simulink model "pe_asm_generator_2"  (R2016b)
settings: Solver=ode23t  StartTime=0.0  StopTime=336  MaxStep=1e-4  RelTol=1e-3  EnableMultiTasking=on
PreLoadFcn:
  | SRated = 150e3; % W
  | VRated = 440; % V
  | FRated = 60; % Hz
  | 
  | QNominal = sin(acos(0.8))*SRated;
  | QPerPhase = QNominal / 3;
  | 
  | IPerPhase = QPerPhase/VRated;
  | Xc = VRated/IPerPhase;
  | reactiveCompensationCapacitance = 1/(2*pi*FRated*Xc);
  | 
  | clear( 'QNominal', 'QPerPhase', 'IPerPhase', 'Xc' );
undefined symbols (not defined in the file or in its folder): pe
libraries: pe_lib x8, nesl_utility x4, fl_lib x2
Description:
  | Three-Phase Asynchronous Wind Turbine Generator
  | 
  | This example shows an induction machine used as a wind turbine generator.
  | The Simple Turbine block converts wind speed to turbine output power by a
  | simple output power versus wind speed characteristic.
  | 
  | When the wind speed is below the cut-in speed or above the cut-out speed,
  | the machine generates zero real power. The machine always consumes
  | reactive power. The Reactive Compensation block offsets the machine's
  | reactive power requirement.
  | 
  | The local load consumes 75kW. The infeed from the power grid meets any
  | wind turbine generation shortfall. When the generator produces more than
  | 75kW, excess power is exported to the grid.
  | 
  | 
  | Copyright 2008-2015 The MathWorks, Inc.
settings Model: Creator=MathWorks  LastModifiedBy=oka
settings DataIOCC: LimitDataPoints=on  SaveFormat=Array  SaveOutput=off  SignalLogging=off  DSMLogging=off  SaveTime=off
settings OptimizationCC: LifeSpan=inf
settings DebuggingCC: UnderspecifiedInitializationDetection=Classic  MergeDetectMultiDrivingBlocksExec=none  SFUnexpectedBacktrackingDiag=warning  SFNoUnconditionalDefaultTransitionDiag=warning  SFExecutionAtInitializationDiag=none
settings HardwareCC: ProdBitPerPointer=32  ProdBitPerSizeT=32  ProdBitPerPtrDiffT=32  ProdLargestAtomicFloat=None  ProdIntDivRoundTo=Undefined  ProdEndianess=Unspecified  ProdWordSize=32  ProdHWDeviceType=32-bit Generic
settings ModelReferenceCC: PropagateSignalLabelsOutOfModel=off
settings GRTTargetCC: TargetLangStandard=C89/C90 (ANSI)  GeneratePreprocessorConditionals=Disable all
settings ConfigComp: CovMetricSettings=dw  CovHtmlReporting=on  CovSaveCumulativeToWorkspaceVar=on  CovSaveSingleToWorkspaceVar=on  CovExternalEMLEnable=off  CovSFcnEnable=off
settings SimscapeCC: SimscapeLogSimulationStatistics=on  SimscapeLogOpenViewer=on  SimscapeLogLimitData=off

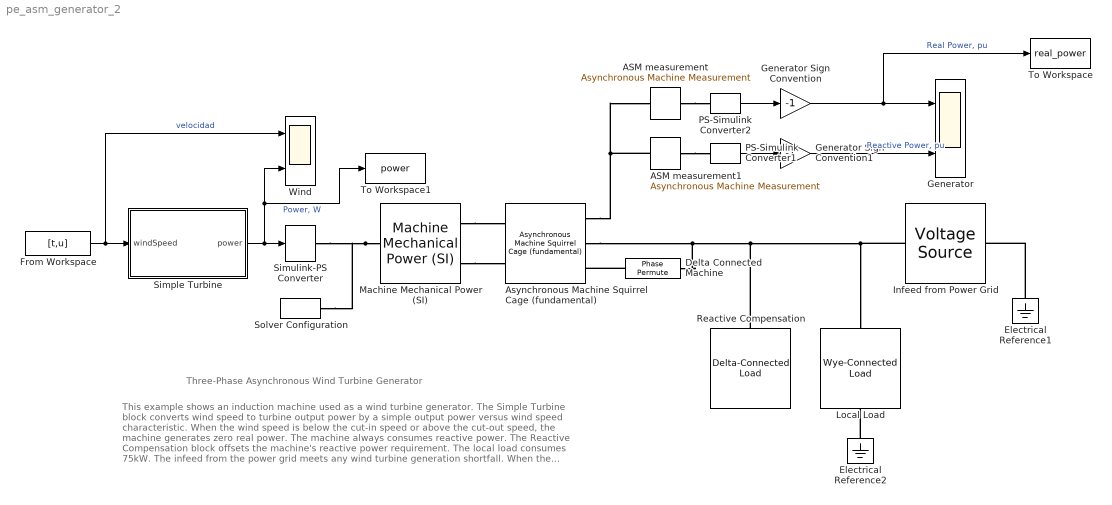
== system pe_asm_generator_2 ==
  note: This example shows an induction machine used as a wind turbine generator.  The Simple
      | Turbine block converts wind speed to turbine output power by a simple output power versus
      | wind speed characteristic.
      | When the wind speed is below the cut-in speed or above the cut-out speed, the machine
      | generates zero real power. The machine always consumes reactive power. The Reactive
      | Compensation block offsets the machine's reactive power requirement.
      | The local load consumes 75kW. The infeed from the power grid meets any wind turbine
      | generation shortfall. When the generator produces more than 75kW, excess power is
      | exported to the grid.
  note: Three-Phase Asynchronous Wind Turbine Generator
  ASM measurement : pe_lib/Machines/Asynchronous Machine Measurement  output_idx=11
  ASM measurement1 : pe_lib/Machines/Asynchronous Machine Measurement  output_idx=12
  Asynchronous Machine Squirrel Cage (fundamental) : pe_lib/Machines/Asynchronous Machine (Squirrel Cage)/Asynchronous Machine Squirrel Cage (fundamental)  SRated=SRated V*A  VRated=VRated V  FRated=FRated Hz  nPolePairs=2  Rs=0.0258  Lls=0.0930  Rrd=0.0145  Llrd=0.0424  Lm=1.7562  L0=0.0930  angular_position0=0 deg  pu_psids0=0  pu_psiqs0=0  pu_psi0s0=0  pu_psidr0=0  pu_psiqr0=0  oneOverOmega=nan s/rad  Lss=nan  Lrrd=nan  shift_3ph=[nan, nan, nan] rad  connection_option=int32(pe.Connection.delta)  base_v=nan V  base_i=nan A  base_torque=nan N*m  base_wMechanical=nan rad/s  base_wElectrical=nan rad/s
  Delta Connected Machine : pe_lib/Connections/Phase Permute
  Electrical Reference1 : fl_lib/Electrical/Electrical Elements/Electrical Reference
  Electrical Reference2 : fl_lib/Electrical/Electrical Elements/Electrical Reference
  From Workspace : FromWorkspace  VariableName=[t,u]  SampleTime=0
  Generator : Scope  NumInputPorts=2
  Generator Sign Convention : Gain  Gain=-1
  Generator Sign Convention1 : Gain  Gain=-1
  Infeed from Power Grid : pe_lib/Sources/Voltage Source  vline_rms=VRated V  shift=0 deg  freq=FRated Hz  harmonic_option=0  harmonic_orders=[5, 7, 11, 13]  harmonic_ratios=[0.1, 0.1, 0.1, 0.1]
  Local Load : pe_lib/Passive Devices/Wye-Connected Load  parameterization=2  component_structure=1  component_structure_PQ=1  R=1 Ohm  L=0.001 H  C=1e-6 F  IL0=[ 0 0 0 ] A  VC0=[ 0 0 0 ] V  R_parasitic=1e-6 Ohm  G_parasitic=1e-6 1/Ohm  VRated=VRated V  FRated=60 Hz  P=75e3 W  Qpos=100 V*A  Qneg=-100 V*A  Vmag0=2.4e+4 V  Vang0=0 deg  Freq0=60 Hz  R_parasitic_PQ=1e-6 Ohm  G_parasitic_PQ=1e-6 1/Ohm
  Machine Mechanical Power (SI) : pe_lib/Machines/Machine Mechanical Power (SI)  power_sign=-1  SRated=SRated V*A  FRated=FRated Hz  nPolePairs=2  torque_factor=2  inertia_option=2  J=27548 kg*m^2  H=4 s*W/V/A  damper_option=2  D=39.0509 N*m/(rad/s)  pu_D=0.01  initialization_option=2  fMechanical0=30 Hz  fElectrical0=FRated Hz
  PS-Simulink Converter1 : nesl_utility/PS-Simulink Converter  PhysicalDomain=network_engine_domain  SubClassName=ps_output  LeftPortType=input  RightPortType=output  PseudoPeriodic=off  Frequencies=[]  Unit=1  AffineConversion=off
  PS-Simulink Converter2 : nesl_utility/PS-Simulink Converter  PhysicalDomain=network_engine_domain  SubClassName=ps_output  LeftPortType=input  RightPortType=output  PseudoPeriodic=off  Frequencies=[]  Unit=1  AffineConversion=off
  Reactive Compensation : pe_lib/Passive Devices/Delta-Connected Load  parameterization=1  component_structure=3  component_structure_PQ=1  R=1 Ohm  L=0.001 H  C=reactiveCompensationCapacitance F  IL0=[ 0 0 0 ] A  VC0=[ 0 0 0 ] V  R_parasitic=1e-6 Ohm  G_parasitic=1e-6 1/Ohm  VRated=2.4e+4 V  FRated=60 Hz  P=1000 W  Qpos=100 V*A  Qneg=-100 V*A  Vmag0=2.4e+4 V  Vang0=0 deg  Freq0=60 Hz  R_parasitic_PQ=1e-6 Ohm  G_parasitic_PQ=1e-6 1/Ohm
  Simple Turbine : MATLAB Function  TreatAsAtomicUnit=on  mask(Simple Turbine){ratedOutputPower=150e3, cutInSpeed=3, ratedOutputSpeed=12, cutOutSpeed=23}
      mask prompts: ratedOutputPower "Rated output power, W"; cutInSpeed "Cut-in speed, m/s"; ratedOutputSpeed "Rated output speed, m/s"; cutOutSpeed "Cut-out speed, m/s"
      mask help:
      | This function implements a simple power versus wind speed characteristic to represent a wind turbine.
      |
      | Given an input of wind speed, m/s, the function outputs turbine power, W.
      |
      | The parameters must meet the following requirement:
      |
      | Cut-in speed < Rated output speed < Cut-out speed
  Simulink-PS Converter : nesl_utility/Simulink-PS Converter  PhysicalDomain=network_engine_domain  SubClassName=ps_input  LeftPortType=input  RightPortType=output  PseudoPeriodic=off  Frequencies=[]  NoiseDistribution=none  NoiseParameters=[]  Unit=1  AffineConversion=off  InputFiltering=off  SimscapeFilterOrder=1  InputFilterTimeConstant=0.001  UdotUserProvided=1
  Solver Configuration : nesl_utility/Solver Configuration  PhysicalDomain=network_engine_domain  SubClassName=solver  LeftPortType=input  RightPortType=generic  Accelerate=off  Tones=[]  Harmonics=[]  SimulateNoise=off  Profile=off  UseLocalSampling=off  EnableSwitchedLinearOptims=on  FrequencyDomain=off  UseCCode=off  RelTol=0.001  AbsTol=1e-06  MinStep=1e-09  ToWorkspace=off  RevertToSquareIcSolve=off  NumHomotopyIterations=100  PhasorMode=off  PhasorModeNumHarmonics=1  OverrideAbsTol=off  DoDC=off  ResidualTolerance=1e-9  UseLocalSolver=on  LocalSolverChoice=NE_BACKWARD_EULER_ADVANCER  LocalSolverSampleTime=1e-3  DoFixedCost=on  MaxNonlinIter=3  MaxModeIter=2  LinearAlgebra=Sparse  DelaysMemoryBudget=1024  AutomaticFiltering=on  FilteringTimeConstant=0.001
  To Workspace : ToWorkspace  VariableName=real_power  SampleTime=-1
  To Workspace1 : ToWorkspace  VariableName=power  SampleTime=-1
  Wind : Scope  NumInputPorts=2
  wires:
  PS-Simulink Converter2/1 -> Generator Sign Convention/1
  PS-Simulink Converter1/1 -> Generator Sign Convention1/1
  Generator Sign Convention/1 -> To Workspace/1, Generator/1  "Real Power, pu"
  Generator Sign Convention1/1 -> Generator/2  "Reactive Power, pu"
  From Workspace/1 -> Simple Turbine/1(windSpeed), Wind/1  "velocidad"
  Simple Turbine/1(power) -> Simulink-PS Converter/1, To Workspace1/1, Wind/2  "Power, W"
  connections:
  Asynchronous Machine Squirrel Cage (fundamental)/RConn2 -- Reactive Compensation/LConn1 -- Infeed from Power Grid/RConn1 -- Local Load/LConn1 -- Delta Connected Machine/LConn1
  Machine Mechanical Power (SI)/RConn1 -- Asynchronous Machine Squirrel Cage (fundamental)/LConn1
  Machine Mechanical Power (SI)/RConn2 -- Asynchronous Machine Squirrel Cage (fundamental)/LConn2
  Machine Mechanical Power (SI)/LConn1 -- Solver Configuration/RConn1 -- Simulink-PS Converter/RConn1
  Asynchronous Machine Squirrel Cage (fundamental)/RConn1 -- ASM measurement1/LConn1 -- ASM measurement/LConn1
  ASM measurement/RConn1 -- PS-Simulink Converter2/LConn1
  Delta Connected Machine/RConn1 -- Asynchronous Machine Squirrel Cage (fundamental)/RConn3
  Electrical Reference1/LConn1 -- Infeed from Power Grid/LConn1
  ASM measurement1/RConn1 -- PS-Simulink Converter1/LConn1
  Electrical Reference2/LConn1 -- Local Load/RConn1

== matlab function pe_asm_generator_2/Simple Turbine ==
  data: windSpeed input; power output; ratedOutputPower parameter; cutInSpeed parameter; ratedOutputSpeed parameter; cutOutSpeed parameter
function power = simpleTurbine( windSpeed, ratedOutputPower, cutInSpeed, ratedOutputSpeed, cutOutSpeed ) %#codegen
%Simple Turbine
% This function implements a simple power versus wind speed characteristic
% to represent a wind turbine.
%
% Given an input of wind speed, m/s, the function outputs turbine power, W.
%
% The parameters must meet the following requirement:
%
% Cut-in speed < Rated output speed < Cut-out speed

% Check rated output power is greater than zero
if ~(ratedOutputPower > 0)
    error( 'Rated output power must be greater than zero.' );
end

% Check cut-in speed is less than rated output speed
if ~(cutInSpeed < ratedOutputSpeed)
    error( 'Cut-in speed must be less than rated output speed.' );
end

% Check rated output speed is less than cut-out speed
if ~(ratedOutputSpeed < cutOutSpeed)
    error( 'Rated output speed must be less than cut-out speed.' );
end

if windSpeed < cutInSpeed
    % Wind speed is less then cut-in speed, power output is zero
    power = 0;
elseif windSpeed < ratedOutputSpeed
    % Wind speed is greater than cut-in speed and less than rated output
    % speed, power output follows linear characteristic from zero to rated
    % power
    cutInGradient = ( ratedOutputPower / ( ratedOutputSpeed - cutInSpeed ) );
    power = cutInGradient * ( windSpeed - cutInSpeed );
elseif windSpeed < cutOutSpeed
    % Wind speed is greater than rated output speed and less than cut-out
    % speed, power output is limited to rated power
    power = ratedOutputPower;
else
    % Wind speed is greater than cut-out speed, power output is zero
    power = 0;
end
